simulink model "Main_simulation"  (R2021b)
settings: Solver=FixedStepAuto  StartTime=0.0  StopTime=Time  FixedStep=t_sample  RelTol=1e-13  AbsTol=1e-19
model workspace (MAT data in the model file):
  S_N = 0
values from neighbouring files (symbols this model uses):
  a = 8.6251e+06    (= 8625100)    [Main.m]    (also in main_code.m)
  A_BN_0 = [1/3, 2/3, 2/3;             2/3, 1/3, -2/3;            -2/3, 2/3,-1/3]    [Main.m]    (also in main_code.m = eye(3))
  A_rw = [1 0 0 1/sqrt(3);         0 1 0 1/sqrt(3) ... (first row only)    [Main.m]    (also in main_code.m)
  A_rw_star = [5/6 -1/6 -1/6;              -1/6  5/6 -1/6 ... (first row only)    [Main.m]    (also in main_code.m)
  acc_m = deg2rad(5)    [main_code.m]
  acc_S = deg2rad(0.25)    [main_code.m]
  c = 299792*10^3    (= 299792000)    [Main.m]    (also in main_code.m)
  control = 2    [main_code.m]
  e = 0.1195    [Main.m]    (also in main_code.m)
  G = 6.67259 * 1e-11    (= 6.67259e-11)    [Main.m]    (also in main_code.m = [gn, gm, gvali, gsvi])
  H = [hn, hm, hvali, hsvi]    [main_code.m]
  i = 0.3815    [Main.m]    (also in main_code.m)
  MB = [2000; 0.3; 1; 0.12].*1e-2    [Main.m]    (also in main_code.m = [1; 0.3; 0.3; 0.3])
  mr = 1.2*1e-4    (= 0.00012)    [Main.m]    (also in main_code.m)
  mu_P = G * Mt    (= 398527110340000)    [main_code.m]
  omega_0 = [om_x, om_y, om_z]    [Main.m]    (also in main_code.m = [w_0x; w_0y; w_0z])
  rho_d_MB = 0.1    [Main.m]    (also in main_code.m)
  rho_d_SP = 0.1    [main_code.m]
  rho_s_MB = 0.5    [Main.m]    (also in main_code.m)
  rho_s_SP = 0.1    [main_code.m]
  sig_b = sig_b^2    [Main.m]    (also in main_code.m)
  sig_n = 0.15*pi/180/3600/sqrt(t_sample)    [Main.m]    (also in main_code.m)
  SP = [2000; 0.3; 1; 0.12].*1e-2    [Main.m]    (also in main_code.m = [3; 0.3; 1; 0.1])
  t_sample = 1/5    (= 0.2)    [Main.m]    (also in main_code.m = 0.1)
  theta0 = 0    [Main.m]
  theta_0 = 0    [main_code.m]
libraries: matrix_library x16, vrlib x8, simulink x2, simulink_extras x1
(part 1 of 4)
settings Model: Creator=adity  LastModifiedBy=adity
settings SolverCC: ZeroCrossControl=DisableAll
settings DebuggingCC: AlgebraicLoopMsg=none

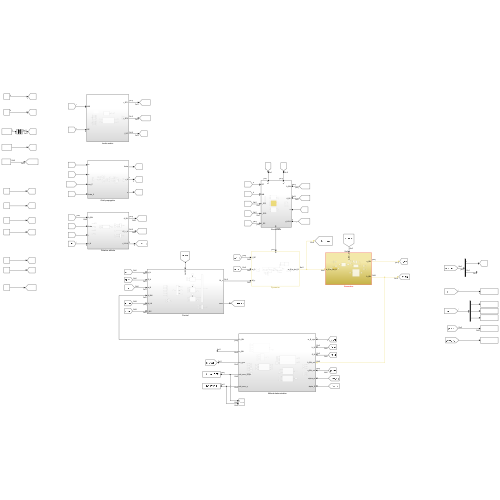
[thumbnail: Simulink's stored preview of the top-level diagram]
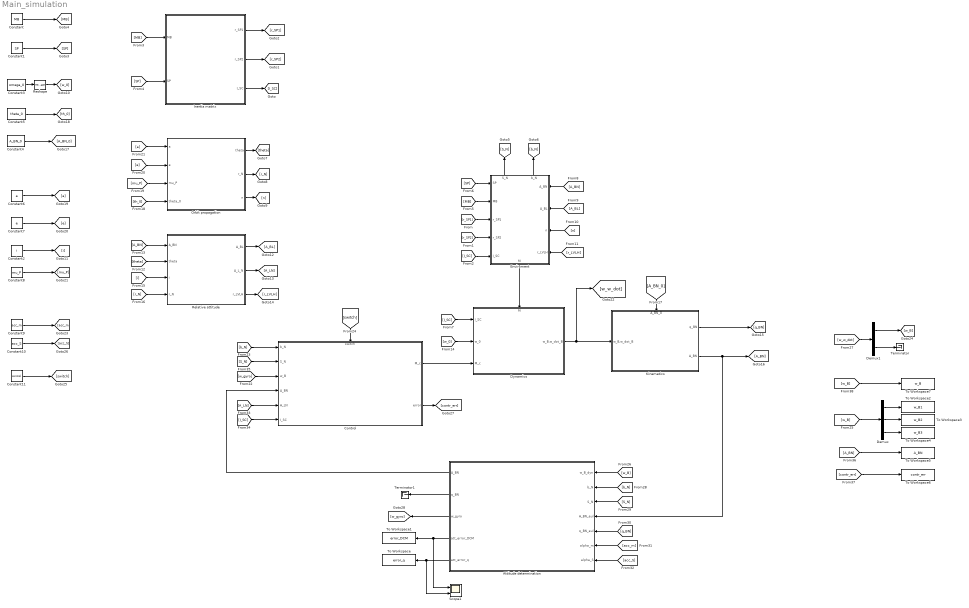
== system Main_simulation ==
  Attitude determination : Subsystem
  Constant : Constant  Value=MB
  Constant1 : Constant  Value=SP
  Constant10 : Constant  Value=acc_S
  Constant11 : Constant  Value=control
  Constant2 : Constant  Value=i
  Constant3 : Constant  Value=omega_0
  Constant4 : Constant  Value=A_BN_0
  Constant5 : Constant  Value=theta_0
  Constant6 : Constant  Value=a
  Constant7 : Constant  Value=e
  Constant8 : Constant  Value=mu_P
  Constant9 : Constant  Value=acc_m
  Control : Subsystem
      settings: PortSchema="{\"entries\":[{\"content\":{\"sides\":[{\"content\":{\"connectorIds\":[\"In1\",\"In2\",\"In3\",\"In4\",\"In5\",\"In6\"]},\"type\":\"ConnectorPlacement.EquallySpacedRectSide\",\"uuid\":\"def4633e-af2e-433f-a30d-e529dfff5b8a\"},{\"content\":{\"connectorIds\":[\"Out1\",\"Out2\"],\"side\":\"RIGHT\"},\"type\":\"ConnectorPlacement.EquallySpacedRectSide\",\"uuid\":\"7f0b35d9-01b3-48bb-a9b6-91939c0c12bf\"},{\"content\":{\"connectorIds\":[\"In7\"],\"side\":\"TOP\"},\"type\":\"ConnectorPlacement.EquallySpacedRectSide\",\"uuid\":\"2761e93e-9101-43c9-a9ad-74672a083719\"}]},\"type\":\"ConnectorPlacement.EquallySpacedConnector\",\"uuid\":\"8d28cc38-98df-4fe9-a975-1ea4168058d4\"}],\"packageUris\":[\"http://schema.mathworks.com/mf0/Connector/R2020b\"],\"version\":\"1.0\"}"
  Demux : Demux  Outputs=3
  Demux1 : Demux  Outputs=2
  Dynamics : Subsystem
      settings: PortSchema="{\"entries\":[{\"content\":{\"sides\":[{\"content\":{\"connectorIds\":[\"In1\",\"In2\",\"In3\"]},\"type\":\"ConnectorPlacement.EquallySpacedRectSide\",\"uuid\":\"0fb0fd28-732a-45b7-951f-4b0b2306202c\"},{\"content\":{\"connectorIds\":[\"Out1\"],\"side\":\"RIGHT\"},\"type\":\"ConnectorPlacement.EquallySpacedRectSide\",\"uuid\":\"160a6d95-5e8b-4088-9ac4-372e2ef53b1e\"},{\"content\":{\"connectorIds\":[\"In4\"],\"side\":\"TOP\"},\"type\":\"ConnectorPlacement.EquallySpacedRectSide\",\"uuid\":\"bc0d773d-9b3c-40c2-804a-fc9efd6e220c\"}]},\"type\":\"ConnectorPlacement.EquallySpacedConnector\",\"uuid\":\"1f85a25c-c8d4-4d9d-9994-483d99135538\"}],\"packageUris\":[\"http://schema.mathworks.com/mf0/Connector/R2020b\"],\"version\":\"1.0\"}"
  Enviroment : Subsystem
      settings: PortSchema="{\"entries\":[{\"content\":{\"sides\":[{\"content\":{\"connectorIds\":[\"Out2\",\"Out3\"]},\"type\":\"ConnectorPlacement.EquallySpacedRectSide\",\"uuid\":\"77a65197-c5ef-4c05-af97-bd670bb59a1b\"},{\"content\":{\"connectorIds\":[\"Out1\"],\"side\":\"RIGHT\"},\"type\":\"ConnectorPlacement.EquallySpacedRectSide\",\"uuid\":\"f4905732-994b-44e8-915f-1f1165b6d340\"},{\"content\":{\"connectorIds\":[\"In1\",\"In2\",\"In3\",\"In4\",\"In5\"],\"side\":\"TOP\"},\"type\":\"ConnectorPlacement.EquallySpacedRectSide\",\"uuid\":\"dbb628bc-072b-4daa-a580-a056bf799753\"},{\"content\":{\"connectorIds\":[\"In6\",\"In7\",\"In8\",\"In9\"],\"side\":\"BOTTOM\"},\"type\":\"ConnectorPlacement.EquallySpacedRectSide\",\"uuid\":\"e6af6235-b92e-4098-9bbc-91b77f168ead\"}]},\"type\":\"ConnectorPlacement.EquallySpacedConnector\",\"uuid\":\"a4645f0d-8f51-4ba7-9ec5-d423e83ccc17\"}],\"packageUris\":[\"http://schema.mathworks.com/mf0/Connector/R2020b\"],\"version\":\"1.0\"}"
  Inertia matrix : Subsystem
  Kinematics : Subsystem
      settings: PortSchema="{\"entries\":[{\"content\":{\"sides\":[{\"content\":{\"connectorIds\":[\"In1\"]},\"type\":\"ConnectorPlacement.EquallySpacedRectSide\",\"uuid\":\"b4580536-f47d-4a76-9d7a-ad9e45e6fd22\"},{\"content\":{\"connectorIds\":[\"Out1\",\"Out2\"],\"side\":\"RIGHT\"},\"type\":\"ConnectorPlacement.EquallySpacedRectSide\",\"uuid\":\"4273ed6e-d469-4a82-9e71-da4fb1c9f709\"},{\"content\":{\"connectorIds\":[\"In2\"],\"side\":\"TOP\"},\"type\":\"ConnectorPlacement.EquallySpacedRectSide\",\"uuid\":\"bac57a2b-a638-4d55-8f6f-550bb52319aa\"}]},\"type\":\"ConnectorPlacement.EquallySpacedConnector\",\"uuid\":\"29527554-7b77-4957-9d93-347c44cffae5\"}],\"packageUris\":[\"http://schema.mathworks.com/mf0/Connector/R2020b\"],\"version\":\"1.0\"}"
  Orbit propagation : Subsystem
  Relative attitude : Subsystem
  Reshape : Reshape  OutputDimensionality=Column vector (2-D)
  Scope1 : Scope  NumInputPorts=2
  Terminator : Terminator
  Terminator1 : Terminator
  To Workspace : ToWorkspace  VariableName=error_q  SaveFormat=Timeseries  SampleTime=-1
  To Workspace1 : ToWorkspace  VariableName=error_DCM  SaveFormat=Timeseries  SampleTime=-1
  To Workspace2 : ToWorkspace  VariableName=w_B1  SaveFormat=Timeseries  SampleTime=-1
  To Workspace3 : ToWorkspace  VariableName=w_B2  SaveFormat=Timeseries  SampleTime=-1
  To Workspace4 : ToWorkspace  VariableName=w_B3  SaveFormat=Timeseries  SampleTime=-1
  To Workspace5 : ToWorkspace  VariableName=A_BN  SaveFormat=Timeseries  SampleTime=-1
  To Workspace6 : ToWorkspace  VariableName=contr_err  SaveFormat=Timeseries  SampleTime=-1
  To Workspace7 : ToWorkspace  VariableName=w_B  SaveFormat=Timeseries  SampleTime=-1
  wires:
  Inertia matrix/3(I_SC) -> [I_SC]
  Inertia matrix/2(r_SP2) -> [r_SP2]
  Inertia matrix/1(r_SP1) -> [r_SP1]
  [r_SP1] -> Enviroment/3(r_SP1)
  [r_SP2] -> Enviroment/4(r_SP2)
  [I_SC] -> Enviroment/5(I_SC)
  Constant/1 -> [MB]
  Constant1/1 -> [SP]
  [MB] -> Inertia matrix/1(MB)
  [SP] -> Inertia matrix/2(SP)
  [MB] -> Enviroment/2(MB)
  [SP] -> Enviroment/1(SP)
  Enviroment/1(M) -> Dynamics/4(M)
  [I_SC] -> Dynamics/1(I_SC)
  Enviroment/2(S_N) -> [S_N]
  Enviroment/3(b_N) -> [b_N]
  [A_BN] -> Enviroment/6(A_BN)
  [A_BL] -> Enviroment/7(A_BL)
  [n] -> Enviroment/8(n)
  [r_LVLH] -> Enviroment/9(r_LVLH)
  Orbit propagation/1(theta) -> [theta]
  Orbit propagation/2(r_N) -> [r_N]
  Orbit propagation/3(n) -> [n]
  [theta] -> Relative attitude/2(theta)
  [A_BN] -> Relative attitude/1(A_BN)
  [w_0] -> Dynamics/2(w_0)
  Constant2/1 -> [i]
  [i] -> Relative attitude/3(i)
  Relative attitude/1(A_BL) -> [A_BL]
  Relative attitude/2(A_L_N) -> [A_LN]
  Dynamics/1(w_B,w_dot_B) -> Kinematics/1(w_B,w_dot_B), [w_w_dot]
  [r_N] -> Relative attitude/4(r_N)
  Relative attitude/3(r_LVLH) -> [r_LVLH]
  Kinematics/1(q_BN) -> [q_BN]
  Kinematics/2(A_BN) -> [A_BN], Attitude determination/4(A_BN_eul)
  [A_BN_0] -> Kinematics/2(A_BN_0)
  Constant4/1 -> [A_BN_0]
  Constant5/1 -> [th_0]
  [th_0] -> Orbit propagation/4(theta_0)
  Constant6/1 -> [a]
  Constant7/1 -> [e]
  Constant8/1 -> [mu_P]
  [mu_P] -> Orbit propagation/3(mu_P)
  [e] -> Orbit propagation/2(e)
  [a] -> Orbit propagation/1(a)
  [w_B] -> Demux/1
  Constant3/1 -> Reshape/1
  Reshape/1 -> [w_0]
  Demux1/1 -> [w_B]
  [w_w_dot] -> Demux1/1
  Demux1/2 -> Terminator/1
  [w_gyro] -> Control/3(w_B)
  [b_N] -> Control/1(b_N)
  [w_B] -> Attitude determination/1(w_B_dyn)
  [b_N] -> Attitude determination/2(b_N)
  [S_N] -> Attitude determination/3(S_N)
  [q_BN] -> Attitude determination/5(q_BN_eul)
  [acc_m] -> Attitude determination/6(alpha_m)
  Constant9/1 -> [acc_m]
  Constant10/1 -> [acc_S]
  [acc_S] -> Attitude determination/7(alpha_S)
  Attitude determination/5(att_error_q) -> Scope1/2, To Workspace/1
  Attitude determination/3(w_gyro) -> [w_gyro]
  [A_LN] -> Control/5(A_LN)
  [I_SC] -> Control/6(I_SC)
  Control/1(M_c) -> Dynamics/3(M_c)
  Demux/1 -> To Workspace2/1
  Demux/2 -> To Workspace3/1
  Demux/3 -> To Workspace4/1
  Constant11/1 -> [switch]
  [switch] -> Control/7(switch)
  Attitude determination/2(q_BN) -> Terminator1/1
  [S_N] -> Control/2(S_N)
  [A_BN] -> To Workspace5/1
  Control/2(error) -> [contr_err]
  [contr_err] -> To Workspace6/1
  [w_B] -> To Workspace7/1
  Attitude determination/1(A_BN) -> Control/4(A_BN)
  Attitude determination/4(att_error_DCM) -> Scope1/1, To Workspace1/1

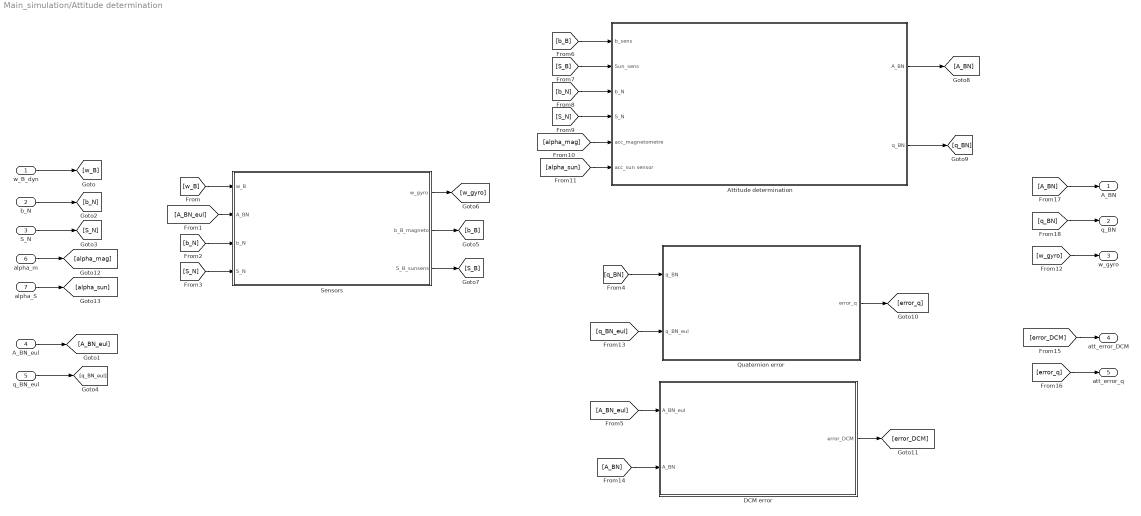
== system Main_simulation/Attitude determination ==
  w_B_dyn : Inport
  b_N : Inport  Port=2
  S_N : Inport  Port=3
  A_BN_eul : Inport  Port=4
  q_BN_eul : Inport  Port=5
  alpha_m : Inport  Port=6
  alpha_S : Inport  Port=7
  Attitude determination : Subsystem
  DCM error : Subsystem
  Quaternion error : Subsystem
  Sensors : Subsystem
  A_BN : Outport
  q_BN : Outport  Port=2
  w_gyro : Outport  Port=3
  att_error_DCM : Outport  Port=4
  att_error_q : Outport  Port=5
  wires:
  w_B_dyn/1 -> [w_B]
  A_BN_eul/1 -> [A_BN_eul]
  b_N/1 -> [b_N]
  S_N/1 -> [S_N]
  [w_B] -> Sensors/1(w_B)
  [A_BN_eul] -> Sensors/2(A_BN)
  [b_N] -> Sensors/3(b_N)
  [S_N] -> Sensors/4(S_N)
  q_BN_eul/1 -> [q_BN_eul]
  Sensors/2(b_B_magneto) -> [b_B]
  Sensors/1(w_gyro) -> [w_gyro]
  Sensors/3(S_B_sunsens) -> [S_B]
  [q_BN] -> Quaternion error/1(q_BN)
  [A_BN_eul] -> DCM error/1(A_BN_eul)
  [b_B] -> Attitude determination/1(b_sens)
  [S_B] -> Attitude determination/2(Sun_sens)
  [b_N] -> Attitude determination/3(b_N)
  [S_N] -> Attitude determination/4(S_N)
  [alpha_mag] -> Attitude determination/5(acc_magnetometre)
  [alpha_sun] -> Attitude determination/6(acc_sun sensor)
  [w_gyro] -> w_gyro/1
  [q_BN_eul] -> Quaternion error/2(q_BN_eul)
  [A_BN] -> DCM error/2(A_BN)
  Quaternion error/1(error_q) -> [error_q]
  DCM error/1(error_DCM) -> [error_DCM]
  [error_DCM] -> att_error_DCM/1
  [error_q] -> att_error_q/1
  [A_BN] -> A_BN/1
  [q_BN] -> q_BN/1
  alpha_m/1 -> [alpha_mag]
  alpha_S/1 -> [alpha_sun]
  Attitude determination/2(q_BN) -> [q_BN]
  Attitude determination/1(A_BN) -> [A_BN]

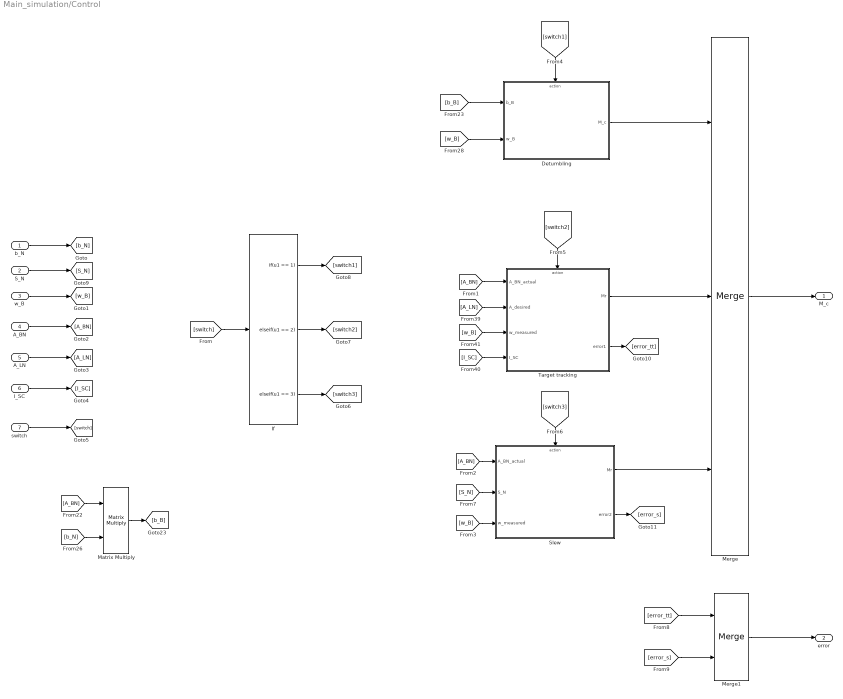
== system Main_simulation/Control ==
  b_N : Inport
  S_N : Inport  Port=2
  w_B : Inport  Port=3
  A_BN : Inport  Port=4
  A_LN : Inport  Port=5
  I_SC : Inport  Port=6
  switch : Inport  Port=7
  Detumbling : Subsystem  TreatAsAtomicUnit=on
  If : If  IfExpression=u1 == 1  ElseIfExpressions=u1 == 2, u1 == 3  ShowElse=off
  Matrix Multiply : Product  Multiplication=Matrix(*)
  Merge : Merge  Inputs=3
  Merge1 : Merge
  Slew : Subsystem  TreatAsAtomicUnit=on
  Target tracking : Subsystem  TreatAsAtomicUnit=on
  M_c : Outport
  error : Outport  Port=2
  wires:
  Matrix Multiply/1 -> [b_B]
  [b_N] -> Matrix Multiply/2
  [A_BN] -> Matrix Multiply/1
  [b_B] -> Detumbling/1(b_B)
  b_N/1 -> [b_N]
  w_B/1 -> [w_B]
  A_BN/1 -> [A_BN]
  Target tracking/1(Mr) -> Merge/2
  [A_LN] -> Target tracking/2(A_desired)
  [A_BN] -> Target tracking/1(A_BN_actual)
  [w_B] -> Target tracking/3(w_measured)
  A_LN/1 -> [A_LN]
  I_SC/1 -> [I_SC]
  [w_B] -> Detumbling/2(w_B)
  Merge/1 -> M_c/1
  Detumbling/1(M_c) -> Merge/1
  [I_SC] -> Target tracking/4(I_SC)
  [A_BN] -> Slew/1(A_BN_actual)
  [w_B] -> Slew/3(w_measured)
  switch/1 -> [switch]
  [switch] -> If/1
  If/3 -> [switch3]
  If/2 -> [switch2]
  If/1 -> [switch1]
  [switch1] -> Detumbling/Action
  [switch2] -> Target tracking/Action
  Slew/1(Mr) -> Merge/3
  S_N/1 -> [S_N]
  [S_N] -> Slew/2(S_N)
  [switch3] -> Slew/Action
  Target tracking/2(error1) -> [error_tt]
  Slew/2(error2) -> [error_s]
  [error_tt] -> Merge1/1
  [error_s] -> Merge1/2
  Merge1/1 -> error/1

== system Main_simulation/Dynamics ==
  I_SC : Inport
  w_0 : Inport  Port=2
  M_c : Inport  Port=3
  M : Inport  Port=4
  Add : Sum
  Cross Product : vrlib/Utilities/Cross Product
  Demux : Demux  Outputs=3
  Gain5 : Gain  Gain=-1
  Integrator4 : Integrator  InitialConditionSource=external  InitialCondition=omega_0
  Mux : Mux  Inputs=2
  Product6 : Product  Multiplication=Matrix(*)
  Product7 : Product  Multiplication=Matrix(*)
  Reciprocal : Product  Inputs=/  Multiplication=Matrix(*)
  Scope : Scope  NumInputPorts=3
  Scope1 : Scope
  Sum2 : Sum
  w_B,w_dot_B : Outport
  wires:
  Sum2/1 -> Product7/2
  Product6/1 -> Cross Product/2
  Product7/1 -> [w_dot_B], Integrator4/1
  Cross Product/1 -> Gain5/1
  Gain5/1 -> Sum2/1
  Integrator4/1 -> [w_B], Demux/1, Cross Product/1, Product6/2
  I_SC/1 -> [I_SC]
  [I_SC] -> Product6/1
  [I_SC] -> Reciprocal/1
  Reciprocal/1 -> Product7/1
  w_0/1 -> [w_0]
  [w_0] -> Integrator4/2
  Demux/2 -> Scope/2  "om_y"
  Demux/1 -> Scope/1  "om_x"
  Demux/3 -> Scope/3  "om_z"
  Add/1 -> Sum2/2
  Mux/1 -> w_B,w_dot_B/1
  [w_B] -> Mux/1
  [w_dot_B] -> Mux/2
  M/1 -> Add/1, Scope1/1
  M_c/1 -> Add/2

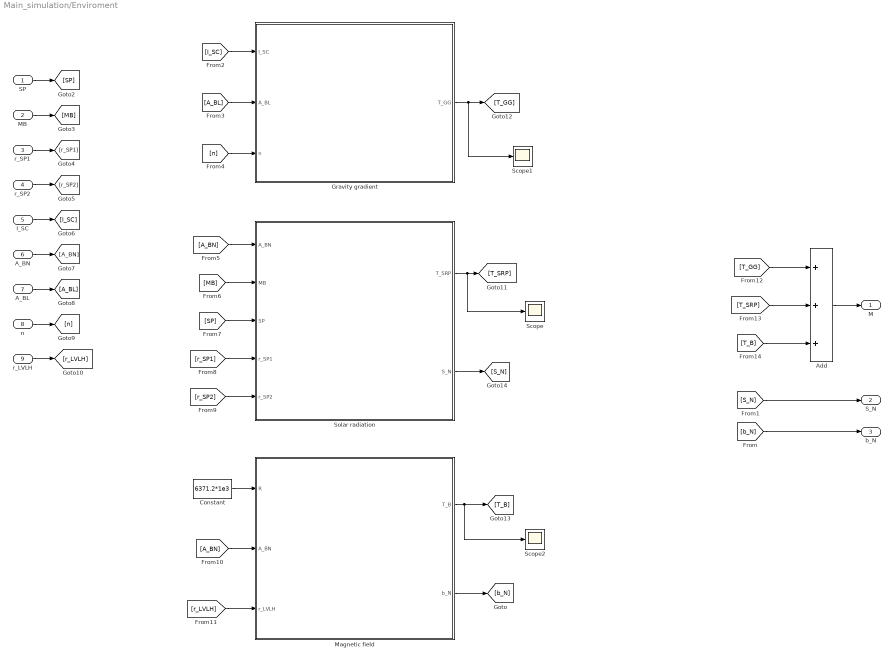
== system Main_simulation/Enviroment ==
  SP : Inport
  MB : Inport  Port=2
  r_SP1 : Inport  Port=3
  r_SP2 : Inport  Port=4
  I_SC : Inport  Port=5
  A_BN : Inport  Port=6
  A_BL : Inport  Port=7
  n : Inport  Port=8
  r_LVLH : Inport  Port=9
  Add : Sum  Inputs=+++
  Constant : Constant  Value=6371.2*1e3
  Gravity gradient : Subsystem
  Magnetic field : Subsystem
  Scope : Scope
  Scope1 : Scope
  Scope2 : Scope
  Solar radiation : Subsystem
  M : Outport
  S_N : Outport  Port=2
  b_N : Outport  Port=3
  wires:
  Add/1 -> M/1
  Constant/1 -> Magnetic field/1(R)
  [b_N] -> b_N/1
  [S_N] -> S_N/1
  SP/1 -> [SP]
  MB/1 -> [MB]
  r_SP1/1 -> [r_SP1]
  r_SP2/1 -> [r_SP2]
  I_SC/1 -> [I_SC]
  A_BN/1 -> [A_BN]
  A_BL/1 -> [A_BL]
  n/1 -> [n]
  r_LVLH/1 -> [r_LVLH]
  Magnetic field/2(b_N) -> [b_N]
  Solar radiation/1(T_SRP) -> Scope/1, [T_SRP]
  Gravity gradient/1(T_GG) -> Scope1/1, [T_GG]
  Magnetic field/1(T_B) -> Scope2/1, [T_B]
  [I_SC] -> Gravity gradient/1(I_SC)
  [A_BL] -> Gravity gradient/2(A_BL)
  [n] -> Gravity gradient/3(n)
  [A_BN] -> Solar radiation/1(A_BN)
  [MB] -> Solar radiation/2(MB)
  [SP] -> Solar radiation/3(SP)
  [r_SP1] -> Solar radiation/4(r_SP1)
  [r_SP2] -> Solar radiation/5(r_SP2)
  [A_BN] -> Magnetic field/2(A_BN)
  [r_LVLH] -> Magnetic field/3(r_LVLH)
  Solar radiation/2(S_N) -> [S_N]
  [T_GG] -> Add/1
  [T_SRP] -> Add/2
  [T_B] -> Add/3

== system Main_simulation/Inertia matrix ==
  note: a long side, b middle side h short side
      | long side on x axis solar panel
      | middle side z axis solar panel
      | long side y axis main body
      | middle side x axis main body
      | short side z axis main body
  MB : Inport
  SP : Inport  Port=2
  Constant : Constant  Value=[19.5 0 0; 0 19 0; 0 0 12.6]  VectorParams1D=off
  Demux : Demux
  Demux1 : Demux
  Reshape : Reshape  OutputDimensionality=Customize  OutputDimensions=[3,3]
  Terminator{,1..5} (6 alike) : Terminator
  r_SP : Subsystem
  r_SP1 : Outport
  r_SP2 : Outport  Port=2
  I_SC : Outport  Port=3
  wires:
  MB/1 -> Demux1/1
  Demux/1 -> Terminator5/1
  r_SP/1(r_SP1) -> [r_SP1]
  [r_SP1] -> r_SP1/1
  [r_SP2] -> r_SP2/1
  r_SP/2(r_SP2) -> [r_SP2]
  Demux/2 -> Terminator4/1
  Demux/3 -> [b_SP]
  Demux/4 -> Terminator3/1
  [b_SP] -> r_SP/1(b_SP)
  Demux1/4 -> Terminator1/1
  Demux1/3 -> Terminator/1
  Demux1/2 -> [a_MB]
  Demux1/1 -> Terminator2/1
  [a_MB] -> r_SP/2(a_MB)
  SP/1 -> Demux/1
  [I_SC] -> I_SC/1
  Constant/1 -> Reshape/1
  Reshape/1 -> [I_SC]

== system Main_simulation/Kinematics ==
  w_B,w_dot_B : Inport
  A_BN_0 : Inport  Port=2
  DCM to quaternion : Subsystem
  Demux : Demux  Outputs=2
  Gain : Gain  Gain=1/2
  Integrator : Integrator  InitialConditionSource=external  InitialCondition=[0; 0; 0; 1]
  Matrix Multiply : Product  Multiplication=Matrix(*)
  Normalisation : Subsystem
  Reshape : Reshape  OutputDimensionality=Column vector (2-D)
  Subsystem : Subsystem
  Terminator : Terminator
  q to DCM : Subsystem
  q_BN : Outport
  A_BN : Outport  Port=2
  wires:
  w_B,w_dot_B/1 -> Demux/1
  Demux/1 -> [w_B]
  Demux/2 -> Terminator/1
  A_BN_0/1 -> [A_BN_0]
  [q_0] -> Integrator/2
  [w_B] -> Subsystem/1(w_B)
  DCM to quaternion/1(q) -> [q_0]
  Subsystem/1(OMEGA) -> [OMEGA]
  Reshape/1 -> Normalisation/1(In1)
  Integrator/1 -> Reshape/1  "q(t)"
  [OMEGA] -> Gain/1
  Gain/1 -> Matrix Multiply/1
  Normalisation/1(Out1) -> Matrix Multiply/2, [q_BN]  "q(t)"
  Matrix Multiply/1 -> Integrator/1  "dq/dt"
  [A_BN_0] -> DCM to quaternion/1(DCM)
  [q_BN] -> q_BN/1
  [A_BN] -> A_BN/1
  q to DCM/1(A_BN) -> [A_BN]
  [q_BN] -> q to DCM/1(q_BN)

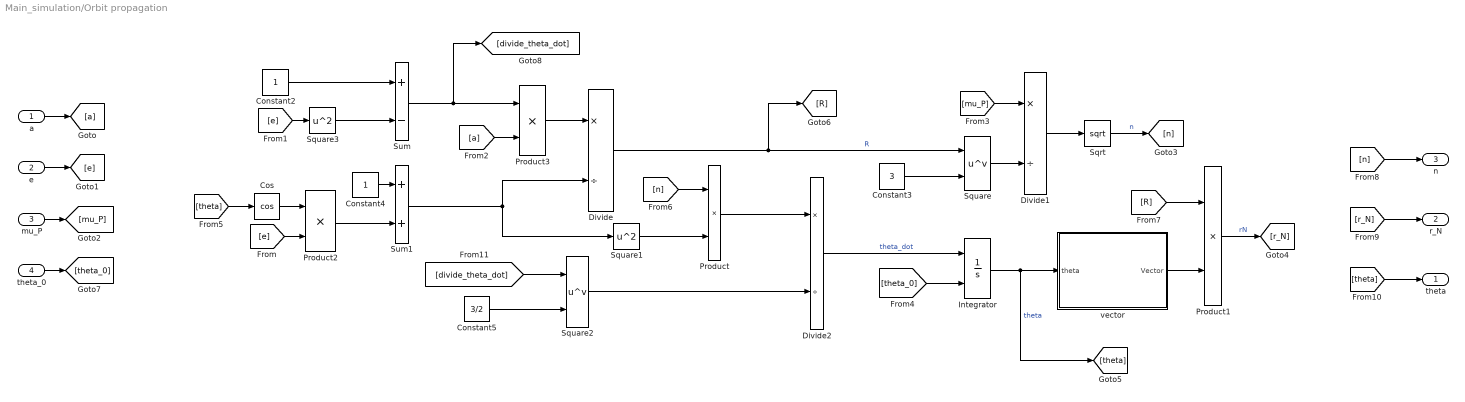
== system Main_simulation/Orbit propagation ==
  a : Inport
  e : Inport  Port=2
  mu_P : Inport  Port=3
  theta_0 : Inport  Port=4
  Constant2 : Constant
  Constant3 : Constant  Value=3
  Constant4 : Constant
  Constant5 : Constant  Value=3/2
  Cos : Trigonometry  Operator=cos
  Divide : Product  Inputs=*/
  Divide1 : Product  Inputs=*/
  Divide2 : Product  Inputs=*/
  Integrator : Integrator  InitialConditionSource=external  InitialCondition=theta0
  Product{,1..3} (4 alike) : Product
  Sqrt : Sqrt  SaturateOnIntegerOverflow=on
  Square : Math  Operator=pow  SaturateOnIntegerOverflow=on
  Square1 : Math  Operator=square  SaturateOnIntegerOverflow=on
  Square2 : Math  Operator=pow  SaturateOnIntegerOverflow=on
  Square3 : Math  Operator=square  SaturateOnIntegerOverflow=on
  Sum : Sum  Inputs=+-
  Sum1 : Sum
  vector : Subsystem
  theta : Outport
  r_N : Outport  Port=2
  n : Outport  Port=3
  wires:
  Constant2/1 -> Sum/1
  Square3/1 -> Sum/2
  Sum/1 -> [divide_theta_dot], Product3/1
  Product3/1 -> Divide/1
  Constant4/1 -> Sum1/1
  Sum1/1 -> Square1/1, Divide/2
  Product2/1 -> Sum1/2
  Cos/1 -> Product2/1
  Integrator/1 -> [theta], vector/1(theta)  "theta"
  Divide1/1 -> Sqrt/1
  [mu_P] -> Divide1/1
  Square/1 -> Divide1/2
  Divide/1 -> [R], Square/1  "R"
  Constant3/1 -> Square/2
  Sqrt/1 -> [n]  "n"
  Square1/1 -> Product/2
  Constant5/1 -> Square2/2
  Product/1 -> Divide2/1
  Divide2/1 -> Integrator/1  "theta_dot"
  vector/1(Vector) -> Product1/2
  Square2/1 -> Divide2/2
  a/1 -> [a]
  e/1 -> [e]
  mu_P/1 -> [mu_P]
  [e] -> Product2/2
  [e] -> Square3/1
  [a] -> Product3/2
  [theta_0] -> Integrator/2
  Product1/1 -> [r_N]  "rN"
  [theta] -> Cos/1
  [n] -> Product/1
  [R] -> Product1/1
  [n] -> n/1
  [r_N] -> r_N/1
  [theta] -> theta/1
  theta_0/1 -> [theta_0]
  [divide_theta_dot] -> Square2/1

== system Main_simulation/Relative attitude ==
  A_BN : Inport
  theta : Inport  Port=2
  i : Inport  Port=3
  r_N : Inport  Port=4
  A_LN : Subsystem
  MatrixMultiply : Product  Multiplication=Matrix(*)
  MatrixMultiply1 : Product  Multiplication=Matrix(*)
  Transpose : Math  Operator=transpose  SaturateOnIntegerOverflow=on
  A_BL : Outport
  A_L_N : Outport  Port=2
  r_LVLH : Outport  Port=3
  wires:
  Transpose/1 -> MatrixMultiply/2
  MatrixMultiply/1 -> A_BL/1  "A_BL"
  theta/1 -> [theta]
  A_BN/1 -> [A_BN]
  [theta] -> A_LN/1(theta)
  A_LN/1(A_L_N) -> [A_LN]
  [i] -> A_LN/2(i)
  i/1 -> [i]
  [A_BN] -> MatrixMultiply/1
  [A_LN] -> Transpose/1
  [A_LN] -> A_L_N/1
  MatrixMultiply1/1 -> r_LVLH/1  "A_BL"
  [A_LN] -> MatrixMultiply1/1
  r_N/1 -> [r_N]
  [r_N] -> MatrixMultiply1/2

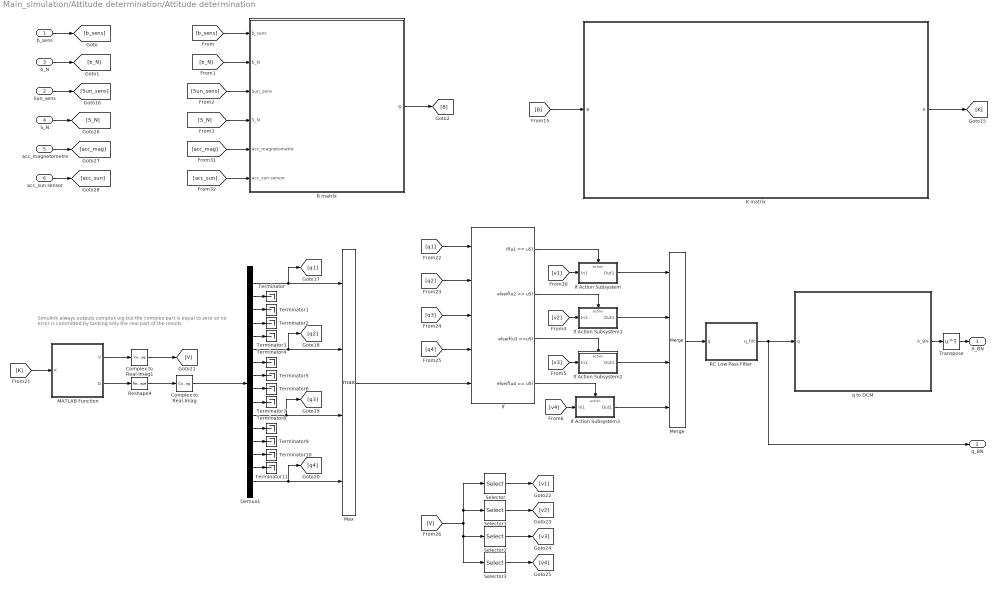
== system Main_simulation/Attitude determination/Attitude determination ==
  note: Simulink always outputs complex eig but the complex part is equal to zero so
      | no error is committed by tanking only the real part of the results
  b_sens : Inport
  Sun_sens : Inport  Port=2
  b_N : Inport  Port=3
  S_N : Inport  Port=4
  acc_magnetometre : Inport  Port=5
  acc_sun sensor : Inport  Port=6
  B matrix : Subsystem
  Complex to Real-Imag : ComplexToRealImag  Output=Real
  Complex to Real-Imag1 : ComplexToRealImag  Output=Real
  Demux1 : Demux  Outputs=16
  If : If  NumInputs=5  IfExpression=u1 == u5  ElseIfExpressions=u2 == u5, u3 ==u5, u4 == u5  ShowElse=off
  If Action Subsystem : Subsystem  TreatAsAtomicUnit=on
  If Action Subsystem1 : Subsystem  TreatAsAtomicUnit=on
  If Action Subsystem2 : Subsystem  TreatAsAtomicUnit=on
  If Action Subsystem3 : Subsystem  TreatAsAtomicUnit=on
  K matrix : Subsystem
  MATLAB Function : MATLAB Function  TreatAsAtomicUnit=on
  Max : MinMax  Function=max  Inputs=4
  Merge : Merge  Inputs=4
  RC Low Pass FIlter : Subsystem
  Reshape4 : Reshape  OutputDimensionality=Column vector (2-D)
  Selector : Selector  NumberOfDimensions=2  InputPortWidth=3  IndexOptions=Index vector (dialog),Index vector (dialog)  Indices=[1 2 3 4],1  OutputSizes=1,1
  Selector1 : Selector  NumberOfDimensions=2  InputPortWidth=3  IndexOptions=Index vector (dialog),Index vector (dialog)  Indices=[1 2 3 4],2  OutputSizes=1,1
  Selector2 : Selector  NumberOfDimensions=2  InputPortWidth=3  IndexOptions=Index vector (dialog),Index vector (dialog)  Indices=[1 2 3 4],3  OutputSizes=1,1
  Selector3 : Selector  NumberOfDimensions=2  InputPortWidth=3  IndexOptions=Index vector (dialog),Index vector (dialog)  Indices=[1 2 3 4],4  OutputSizes=1,1
  Terminator{,1..11} (12 alike) : Terminator
  Transpose : Math  Operator=transpose  SaturateOnIntegerOverflow=on
  q to DCM : Subsystem
  A_BN : Outport
  q_BN : Outport  Port=2
  wires:
  MATLAB Function/2(D) -> Reshape4/1
  Demux1/2 -> Terminator/1
  Demux1/3 -> Terminator1/1
  Demux1/4 -> Terminator2/1
  Demux1/5 -> Terminator3/1
  Demux1/6 -> [q2], Max/2
  Demux1/7 -> Terminator4/1
  Demux1/8 -> Terminator5/1
  Demux1/9 -> Terminator6/1
  Demux1/10 -> Terminator7/1
  Demux1/11 -> [q3], Max/3
  Demux1/16 -> [q4], Max/4
  Demux1/12 -> Terminator8/1
  Demux1/13 -> Terminator9/1
  Demux1/14 -> Terminator10/1
  Demux1/15 -> Terminator11/1
  Reshape4/1 -> Complex to Real-Imag/1
  Max/1 -> If/5
  Demux1/1 -> [q1], Max/1
  [q1] -> If/1
  [q2] -> If/2
  [q4] -> If/4
  [q3] -> If/3
  MATLAB Function/1(V) -> Complex to Real-Imag1/1
  Selector1/1 -> [v2]
  Selector3/1 -> [v4]
  Selector2/1 -> [v3]
  Selector/1 -> [v1]
  [V] -> Selector/1, Selector1/1, Selector3/1, Selector2/1
  If/1 -> If Action Subsystem/Action
  If Action Subsystem/1(Out1) -> Merge/1
  If Action Subsystem3/1(Out1) -> Merge/4
  If Action Subsystem2/1(Out1) -> Merge/3
  If Action Subsystem1/1(Out1) -> Merge/2
  [v1] -> If Action Subsystem/1(In1)
  Complex to Real-Imag/1 -> Demux1/1
  Complex to Real-Imag1/1 -> [V]
  [K] -> MATLAB Function/1(K)
  B matrix/1(B) -> [B]
  b_N/1 -> [b_N]
  S_N/1 -> [S_N]
  acc_magnetometre/1 -> [acc_mag]
  acc_sun sensor/1 -> [acc_sun]
  [b_sens] -> B matrix/1(b_sens)
  [b_N] -> B matrix/2(b_N)
  [Sun_sens] -> B matrix/3(Sun_sens)
  [S_N] -> B matrix/4(S_N)
  [acc_mag] -> B matrix/5(acc_magnetometre)
  [acc_sun] -> B matrix/6(acc_sun sensor)
  [B] -> K matrix/1(B)
  K matrix/1(K) -> [K]
  Sun_sens/1 -> [Sun_sens]
  b_sens/1 -> [b_sens]
  q to DCM/1(A_BN) -> Transpose/1
  Merge/1 -> RC Low Pass FIlter/1(q)
  [v2] -> If Action Subsystem1/1(In1)
  If/2 -> If Action Subsystem1/Action
  If/3 -> If Action Subsystem2/Action
  [v3] -> If Action Subsystem2/1(In1)
  [v4] -> If Action Subsystem3/1(In1)
  If/4 -> If Action Subsystem3/Action
  RC Low Pass FIlter/1(q_filt) -> q_BN/1, q to DCM/1(q)
  Transpose/1 -> A_BN/1

== system Main_simulation/Attitude determination/DCM error ==
  A_BN_eul : Inport
  A_BN : Inport  Port=2
  Add : Sum  Inputs=+-
  Constant : Constant  Value=[1 0 0; 0 1 0; 0 0 1]
  Matrix Multiply : Product  Multiplication=Matrix(*)
  Reshape : Reshape  OutputDimensionality=Customize  OutputDimensions=[3,3]
  Transpose : Math  Operator=transpose  SaturateOnIntegerOverflow=on
  error_DCM : Outport
  wires:
  A_BN_eul/1 -> Transpose/1
  Transpose/1 -> Matrix Multiply/2
  A_BN/1 -> Matrix Multiply/1
  Add/1 -> error_DCM/1
  Matrix Multiply/1 -> Add/1
  Constant/1 -> Reshape/1
  Reshape/1 -> Add/2

== system Main_simulation/Attitude determination/Quaternion error ==
  q_BN : Inport
  q_BN_eul : Inport  Port=2
  Matrix Multiply : Product  Multiplication=Matrix(*)
  Q matrix : Subsystem
  q_vect : Selector  InputPortWidth=4  IndexOptions=Index vector (dialog)  Indices=[1 2 3]  OutputSizes=1
  error_q : Outport
  wires:
  q_BN/1 -> [q_att]
  q_BN_eul/1 -> [q_eul]
  [q_eul] -> Q matrix/1(q_eul)
  [q_att] -> Matrix Multiply/2
  Q matrix/1(Q_eul) -> Matrix Multiply/1
  Matrix Multiply/1 -> q_vect/1
  q_vect/1 -> error_q/1

== system Main_simulation/Attitude determination/Sensors ==
  w_B : Inport
  A_BN : Inport  Port=2
  b_N : Inport  Port=3
  S_N : Inport  Port=4
  Gyroscopes : Subsystem
  Magnetometer : Subsystem
  Sun sensor : Subsystem
  Zero-Order Hold{,1..3} (4 alike) : ZeroOrderHold  SampleTime=t_sample
  w_gyro : Outport
  b_B_magneto : Outport  Port=2
  S_B_sunsens : Outport  Port=3
  wires:
  [w_B] -> Gyroscopes/1(omega)
  [A_BN] -> Magnetometer/1(A_BN)
  [A_BN] -> Sun sensor/2(A_BN)
  Gyroscopes/1(w_gyro) -> [w_gyro]
  Magnetometer/1(b_B) -> [b_B]
  Sun sensor/1(S_B) -> [S_B]
  [w_gyro] -> w_gyro/1
  [b_B] -> b_B_magneto/1
  [S_B] -> S_B_sunsens/1
  w_B/1 -> Zero-Order Hold/1
  A_BN/1 -> Zero-Order Hold1/1
  b_N/1 -> Zero-Order Hold2/1
  S_N/1 -> Zero-Order Hold3/1
  [S_N] -> Sun sensor/1(S_N)
  [b_N] -> Magnetometer/2(b_N)
  Zero-Order Hold/1 -> [w_B]
  Zero-Order Hold1/1 -> [A_BN]
  Zero-Order Hold2/1 -> [b_N]
  Zero-Order Hold3/1 -> [S_N]

== system Main_simulation/Control/Detumbling ==
  b_B : Inport
  w_B : Inport  Port=2
  Action Port : ActionPort  ActionPortLabel=if(u1 == 1)
  Cross Product : matrix_library/Cross Product
      settings: SourceProductBaseCode=SL
  Cross Product1 : matrix_library/Cross Product
      settings: SourceProductBaseCode=SL
  Divide : Product  Inputs=/*
  Dot Product : DotProduct  InputSameDT=on  OutDataTypeStr=Inherit: Inherit via internal rule
  Gain : Gain  Gain=-1
  Product : Product
  k : Constant  Value=3.5e-2
  M_c : Outport
  wires:
  [b_B] -> Dot Product/2, Dot Product/1
  Product/1 -> Cross Product1/1
  Gain/1 -> Product/2
  Dot Product/1 -> Divide/1
  Divide/1 -> Product/1
  [b_B] -> Cross Product1/2
  b_B/1 -> [b_B]
  Cross Product/1 -> Divide/2
  [b_B] -> Cross Product/1
  w_B/1 -> [w_B]
  k/1 -> Gain/1
  Cross Product1/1 -> M_c/1
  [w_B] -> Cross Product/2

== system Main_simulation/Control/Slew ==
  A_BN_actual : Inport
  S_N : Inport  Port=2
  w_measured : Inport  Port=3
  Action Port : ActionPort  ActionPortLabel=elseif( u1 == 3)
  Demux : Demux  Outputs=3
  Desired attitude : Subsystem
  Gain : Gain  Gain=-1
  Gain1 : Gain  Gain=-1
  Matrix Multiply : Product  Multiplication=Matrix(*)
  Mux : Mux  Inputs=3
  Product : Product
  Product1 : Product
  Reaction wheel : Subsystem
  Reshape : Reshape  OutputDimensionality=Customize  OutputDimensions=[3,1]
  Reshape1 : Reshape  OutputDimensionality=Column vector (2-D)
  Reshape2 : Reshape  OutputDimensionality=Column vector (2-D)
  Scope{,1..3} (4 alike) : Scope
  Selector : Selector  NumberOfDimensions=2  InputPortWidth=3  IndexOptions=Index vector (dialog),Index vector (dialog)  Indices=2,1  OutputSizes=1,1
  Selector1 : Selector  NumberOfDimensions=2  InputPortWidth=3  IndexOptions=Index vector (dialog),Index vector (dialog)  Indices=3,1  OutputSizes=1,1
  Selector2 : Selector  NumberOfDimensions=2  InputPortWidth=3  IndexOptions=Index vector (dialog),Index vector (dialog)  Indices=3,2  OutputSizes=1,1
  Sum : Sum  Inputs=|+|-|
  Sum1 : Sum  Inputs=|+|+|
  Terminator : Terminator
  Terminator1 : Terminator
  Transpose : Math  Operator=transpose  SaturateOnIntegerOverflow=on
  Transpose1 : Math  Operator=transpose  SaturateOnIntegerOverflow=on
  k1 : Constant  Value=9.99e-2
  k2 : Constant  Value=1.25e-3
  Mr : Outport
  error2 : Outport  Port=2
  wires:
  Product/1 -> Reshape1/1
  Transpose1/1 -> Sum/1
  Selector1/1 -> Mux/2
  Reshape2/1 -> Sum1/1
  Sum/1 -> Selector1/1, Selector/1, Selector2/1
  Demux/3 -> Terminator1/1
  Selector2/1 -> Mux/3
  Matrix Multiply/1 -> Transpose1/1, Sum/2
  k2/1 -> Gain/1
  Reshape1/1 -> Sum1/2
  Mux/1 -> Reshape/1, Demux/1, Scope/1
  Sum1/1 -> Reaction wheel/1(Mc), Scope2/1
  k1/1 -> Gain1/1
  Product1/1 -> Reshape2/1
  Transpose/1 -> Matrix Multiply/2
  Gain1/1 -> Product/2
  Selector/1 -> Mux/1
  Demux/1 -> error2/1
  Reshape/1 -> Product1/1
  Demux/2 -> Terminator/1
  Gain/1 -> Product1/2
  Reaction wheel/1(Mr) -> Mr/1
  [w_B] -> Reaction wheel/2(w)
  A_BN_actual/1 -> [A_BN]
  [A_BN] -> Matrix Multiply/1
  [A_BN] -> Scope1/1
  Desired attitude/1(Desired A_BN) -> Transpose/1
  S_N/1 -> [S_N]
  w_measured/1 -> [w_B]
  [w_B] -> Scope3/1
  [w_B] -> Product/1
  [S_N] -> Desired attitude/1(S_N)

== system Main_simulation/Control/Target tracking ==
  A_BN_actual : Inport
  A_desired : Inport  Port=2
  w_measured : Inport  Port=3
  I_SC : Inport  Port=4
  Action Port : ActionPort  ActionPortLabel=elseif(u1 == 2)
  Cross Product : matrix_library/Cross Product
      settings: SourceProductBaseCode=SL
  Demux : Demux  Outputs=3
  Gain : Gain  Gain=-1
  Gain1 : Gain  Gain=-1
  Matrix Multiply : Product  Multiplication=Matrix(*)
  Matrix Multiply1 : Product  Multiplication=Matrix(*)
  Mux : Mux  Inputs=3
  Product : Product
  Product1 : Product
  Reaction wheel : Subsystem
  Reshape : Reshape  OutputDimensionality=Customize  OutputDimensions=[3,1]
  Reshape1 : Reshape  OutputDimensionality=Column vector (2-D)
  Reshape2 : Reshape  OutputDimensionality=Column vector (2-D)
  Scope : Scope
  Scope1 : Scope
  Scope4 : Scope
  Selector : Selector  NumberOfDimensions=2  InputPortWidth=3  IndexOptions=Index vector (dialog),Index vector (dialog)  Indices=2,1  OutputSizes=1,1
  Selector1 : Selector  NumberOfDimensions=2  InputPortWidth=3  IndexOptions=Index vector (dialog),Index vector (dialog)  Indices=3,1  OutputSizes=1,1
  Selector2 : Selector  NumberOfDimensions=2  InputPortWidth=3  IndexOptions=Index vector (dialog),Index vector (dialog)  Indices=3,2  OutputSizes=1,1
  Sum : Sum  Inputs=|+|-|
  Sum1 : Sum  Inputs=|+|+|+|
  Terminator : Terminator
  Terminator1 : Terminator
  Transpose : Math  Operator=transpose  SaturateOnIntegerOverflow=on
  Transpose1 : Math  Operator=transpose  SaturateOnIntegerOverflow=on
  k1 : Constant  Value=9.99e-2
  k2 : Constant  Value=1.5e-3
  Mr : Outport
  error1 : Outport  Port=2
  wires:
  Demux/1 -> error1/1
  Mux/1 -> Scope/1, Demux/1, Reshape/1
  A_BN_actual/1 -> Scope1/1, Matrix Multiply/1
  w_measured/1 -> [w_B]
  I_SC/1 -> [I_mat]
  Demux/3 -> Terminator1/1
  Matrix Multiply1/1 -> Cross Product/2
  Product/1 -> Reshape1/1
  Cross Product/1 -> Sum1/3
  k2/1 -> Gain/1
  k1/1 -> Gain1/1
  Matrix Multiply/1 -> Sum/2, Transpose1/1
  [I_mat] -> Matrix Multiply1/1
  Gain/1 -> Product1/2
  Reshape1/1 -> Sum1/2
  Transpose/1 -> Matrix Multiply/2
  Reshape/1 -> Product1/1
  Selector1/1 -> Mux/2
  Selector2/1 -> Mux/3
  Reshape2/1 -> Sum1/1
  Demux/2 -> Terminator/1
  A_desired/1 -> Scope4/1, Transpose/1
  Sum/1 -> Selector2/1, Selector/1, Selector1/1
  Transpose1/1 -> Sum/1
  Selector/1 -> Mux/1
  Gain1/1 -> Product/2
  Product1/1 -> Reshape2/1
  [w_B] -> Reaction wheel/2(w)
  Sum1/1 -> Reaction wheel/1(Mc)
  Reaction wheel/1(Mr) -> Mr/1
  [w_B] -> Product/1
  [w_B] -> Matrix Multiply1/2
  [w_B] -> Cross Product/1

== system Main_simulation/Enviroment/Gravity gradient ==
  I_SC : Inport
  A_BL : Inport  Port=2
  n : Inport  Port=3
  Constant : Constant  Value=3
  Constant1 : Constant  Value=[1 0 0]
  Demux : Demux  Outputs=9
  Demux1 : Demux  Outputs=3
  Matrix Multiply : Product  Multiplication=Matrix(*)
  Mux : Mux  Inputs=3
  Product{,1..9} (10 alike) : Product
  Reshape : Reshape  OutputDimensionality=Column vector (2-D)
  Reshape1 : Reshape  OutputDimensionality=Column vector (2-D)
  Reshape2 : Reshape  OutputDimensionality=Column vector (2-D)
  Scope : Scope  NumInputPorts=3
  Square : Math  Operator=square  SaturateOnIntegerOverflow=on
  Sum : Sum  Inputs=+-
  Sum1 : Sum  Inputs=+-
  Sum2 : Sum  Inputs=+-
  Terminator{,1..5} (6 alike) : Terminator
  T_GG : Outport
  wires:
  Demux/4 -> Terminator2/1
  Demux1/1 -> Product5/2, Product7/2
  Demux/2 -> Terminator/1
  Product6/1 -> Product9/1
  Sum/1 -> Product1/1
  Product1/1 -> Product6/1
  Demux/7 -> Terminator4/1
  Demux1/3 -> Product6/2, Product8/2
  Demux/1 -> Sum1/1
  Product5/1 -> Product8/1
  Demux/3 -> Terminator1/1
  I_SC/1 -> Reshape1/1
  Matrix Multiply/1 -> Demux1/1
  Demux/9 -> Sum2/2, Sum1/2, Sum/1
  Constant1/1 -> Reshape/1
  Sum1/1 -> Product2/1
  Sum2/1 -> Product3/1
  Product7/1 -> Scope/3, Mux/3
  Mux/1 -> Reshape2/1
  Demux/5 -> Sum/2, Sum2/1
  Demux/8 -> Terminator5/1
  A_BL/1 -> Matrix Multiply/1
  Product4/1 -> Product7/1
  Product8/1 -> Scope/2, Mux/2
  Demux/6 -> Terminator3/1
  Demux1/2 -> Product4/2, Product9/2
  Product2/1 -> Product5/1
  Product9/1 -> Scope/1, Mux/1
  Product3/1 -> Product4/1
  Reshape/1 -> Matrix Multiply/2
  Reshape1/1 -> Demux/1
  Reshape2/1 -> T_GG/1
  Square/1 -> Product/1
  Product/1 -> Product2/2, Product1/2, Product3/2
  Constant/1 -> Product/2
  n/1 -> Square/1

== system Main_simulation/Enviroment/Magnetic field ==
  R : Inport
  A_BN : Inport  Port=2
  r_LVLH : Inport  Port=3
  Cross Product : matrix_library/Cross Product
      settings: SourceProductBaseCode=SL
  b_B : Subsystem
  parasitic torque : Subsystem
  T_B : Outport
  b_N : Outport  Port=2
  wires:
  parasitic torque/1(m_par) -> [m_par]
  b_B/1(b_B) -> [b_B]
  b_B/2(b_N) -> [b_N]
  [m_par] -> Cross Product/1
  [b_B] -> Cross Product/2
  [b_N] -> b_N/1
  A_BN/1 -> [A_BN]
  R/1 -> [R]
  r_LVLH/1 -> [r_LVLH]
  [A_BN] -> b_B/1(A_BN)
  [R] -> b_B/2(R)
  [r_LVLH] -> b_B/3(r_LVLH)
  Cross Product/1 -> T_B/1

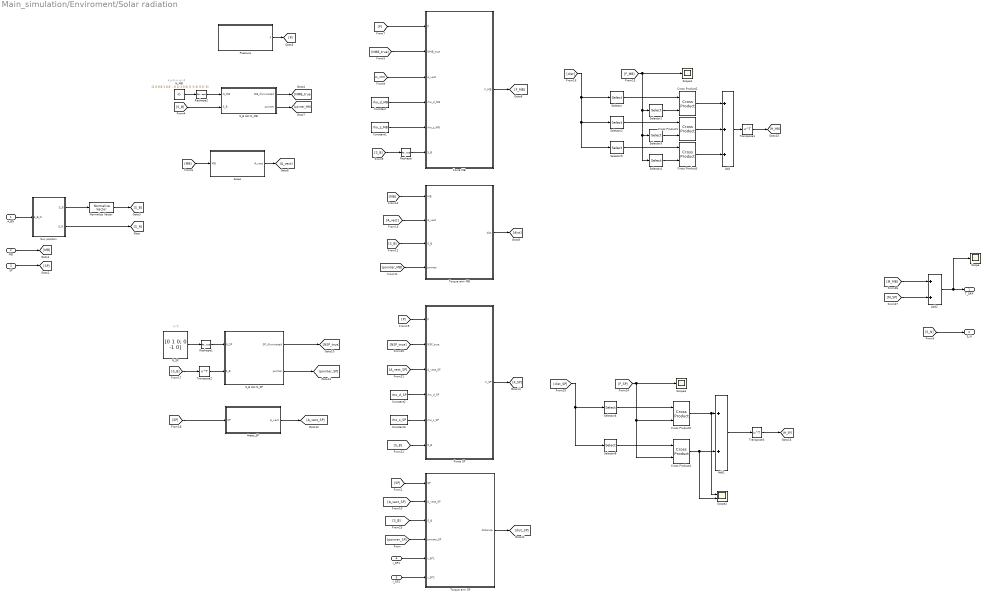
== system Main_simulation/Enviroment/Solar radiation ==
  note: x,y,z,-x,-y,-z
  note: y,-y
  A_BN : Inport
  MB : Inport  Port=2
  SP : Inport  Port=3
  r_SP1 : Inport  Port=4
  r_SP2 : Inport  Port=5
  Add : Sum  Inputs=3
  Add1 : Sum
  Add2 : Sum
  Areas : Subsystem
  Areas_SP : Subsystem
  Constant : Constant  Value=rho_d_MB
  Constant1 : Constant  Value=rho_s_MB
  Constant2 : Constant  Value=rho_d_SP
  Constant3 : Constant  Value=rho_s_SP
  Cross Product{1..5} (5 alike) : matrix_library/Cross Product
      settings: SourceProductBaseCode=SL
  Force MB : Subsystem
  Force SP : Subsystem
  N_MB : Constant  Value=[1 0 0;0 1 0;0 0 1;-1 0 0; 0 -1 0; 0 0 -1]  VectorParams1D=off
  N_SP : Constant  Value=[0 1 0; 0 -1 0]  VectorParams1D=off
  Normalize Vector : vrlib/Utilities/Normalize Vector  maxzero=0
  Pressure : Subsystem
  Reshape : Reshape  OutputDimensionality=Column vector (2-D)
  Reshape1 : Reshape  OutputDimensionality=Customize  OutputDimensions=[2,3]
  Reshape2 : Reshape  OutputDimensionality=Customize  OutputDimensions=[6,3]
  S_B dot N_MB : Subsystem
  S_B dot N_SP : Subsystem
  Scope : Scope
  Scope1 : Scope
  Scope2 : Scope  NumInputPorts=2
  Scope3 : Scope
  Selector : Selector  NumberOfDimensions=2  InputPortWidth=3  IndexOptions=Index vector (dialog),Index vector (dialog)  Indices=1,[1 2 3]  OutputSizes=1,1
  Selector1 : Selector  NumberOfDimensions=2  InputPortWidth=3  IndexOptions=Index vector (dialog),Index vector (dialog)  Indices=1,[1 2 3]  OutputSizes=1,1
  Selector2 : Selector  NumberOfDimensions=2  InputPortWidth=3  IndexOptions=Index vector (dialog),Index vector (dialog)  Indices=2,[1 2 3]  OutputSizes=1,1
  Selector3 : Selector  NumberOfDimensions=2  InputPortWidth=3  IndexOptions=Index vector (dialog),Index vector (dialog)  Indices=2,[1 2 3]  OutputSizes=1,1
  Selector4 : Selector  NumberOfDimensions=2  InputPortWidth=3  IndexOptions=Index vector (dialog),Index vector (dialog)  Indices=3,[1 2 3]  OutputSizes=1,1
  Selector5 : Selector  NumberOfDimensions=2  InputPortWidth=3  IndexOptions=Index vector (dialog),Index vector (dialog)  Indices=3,[1 2 3]  OutputSizes=1,1
  Selector6 : Selector  NumberOfDimensions=2  InputPortWidth=3  IndexOptions=Index vector (dialog),Index vector (dialog)  Indices=1,[1 2 3]  OutputSizes=1,1
  Selector8 : Selector  NumberOfDimensions=2  InputPortWidth=3  IndexOptions=Index vector (dialog),Index vector (dialog)  Indices=2,[1 2 3]  OutputSizes=1,1
  Sun position : Subsystem
  Torque arm MB : Subsystem
  Torque arm SP : Subsystem
  Transpose1 : Math  Operator=transpose  SaturateOnIntegerOverflow=on
  Transpose2 : Math  Operator=transpose  SaturateOnIntegerOverflow=on
  Transpose3 : Math  Operator=transpose  SaturateOnIntegerOverflow=on
  T_SRP : Outport
  S_N : Outport  Port=2
  wires:
  A_BN/1 -> Sun position/1(A_B_N)
  Sun position/1(S_B) -> Normalize Vector/1
  Normalize Vector/1 -> [S_B]
  r_SP1/1 -> Torque arm SP/5(r_SP1)
  r_SP2/1 -> Torque arm SP/6(r_SP2)
  MB/1 -> [MB]
  SP/1 -> [SP]
  Sun position/2(S_N) -> [S_N]
  [S_N] -> S_N/1
  N_MB/1 -> Reshape2/1
  S_B dot N_MB/1(MB_illuminated) -> [NMB_true]
  [NMB_true] -> Force MB/2(NMB_true)
  [S_B] -> S_B dot N_MB/2(S_B)
  [MB] -> Areas/1(MB)
  Pressure/1(P) -> [P]
  Areas/1(A_vect) -> [A_vect]
  [P] -> Force MB/1(P)
  [A_vect] -> Force MB/3(A_vect)
  Constant/1 -> Force MB/4(rho_d_MB)
  Constant1/1 -> Force MB/5(rho_s_MB)
  [S_B] -> Reshape/1
  S_B dot N_MB/2(pointer) -> [pointer_MB]
  [pointer_MB] -> Torque arm MB/4(pointer)
  [S_B] -> Torque arm MB/3(S_B)
  [A_vect] -> Torque arm MB/2(A_vect)
  [MB] -> Torque arm MB/1(MB)
  Reshape/1 -> Force MB/6(S_B)
  Cross Product2/1 -> Add/1
  Selector/1 -> Cross Product2/1
  Selector1/1 -> Cross Product2/2
  Selector3/1 -> Cross Product1/2
  Selector2/1 -> Cross Product1/1
  [dist] -> Selector2/1, Selector5/1, Selector/1
  Cross Product1/1 -> Add/2
  Force MB/1(F_MB) -> [F_MB]
  [F_MB] -> Scope1/1, Selector4/1, Selector3/1, Selector1/1
  Cross Product3/1 -> Add/3
  Selector4/1 -> Cross Product3/2
  Selector5/1 -> Cross Product3/1
  Add/1 -> Transpose1/1
  Torque arm MB/1(dist) -> [dist]
  S_B dot N_SP/2(pointer) -> [pointer_SP]
  Areas_SP/1(A_vect) -> [A_vect_SP]
  [SP] -> Areas_SP/1(SP)
  Transpose2/1 -> S_B dot N_SP/2(S_B)
  [S_B] -> Transpose2/1
  S_B dot N_SP/1(SP_illuminated) -> [NSP_true]
  N_SP/1 -> Reshape1/1
  Reshape1/1 -> S_B dot N_SP/1(N_SP)
  Reshape2/1 -> S_B dot N_MB/1(N_MB)
  [P] -> Force SP/1(P)
  [NSP_true] -> Force SP/2(NSP_true)
  [A_vect_SP] -> Force SP/3(A_vect_SP)
  Constant2/1 -> Force SP/4(rho_d_SP)
  Constant3/1 -> Force SP/5(rho_s_SP)
  [S_B] -> Force SP/6(S_B)
  [pointer_SP] -> Torque arm SP/4(pointer_SP)
  [SP] -> Torque arm SP/1(SP)
  [A_vect_SP] -> Torque arm SP/2(A_vect_SP)
  [S_B] -> Torque arm SP/3(S_B)
  Torque arm SP/1(distance) -> [dist_SP]
  Force SP/1(F_SP) -> [F_SP]
  Transpose3/1 -> [M_SP]
  Add1/1 -> Transpose3/1
  Cross Product4/1 -> Scope2/2, Add1/2
  [dist_SP] -> Selector6/1, Selector8/1
  Selector8/1 -> Cross Product4/1
  [F_SP] -> Cross Product5/2, Cross Product4/2, Scope3/1
  Selector6/1 -> Cross Product5/1
  Cross Product5/1 -> Scope2/1, Add1/1
  Transpose1/1 -> [M_MB]
  [M_MB] -> Add2/1
  Add2/1 -> Scope/1, T_SRP/1
  [M_SP] -> Add2/2

== system Main_simulation/Inertia matrix/r_SP ==
  b_SP : Inport
  a_MB : Inport  Port=2
  Constant : Constant  Value=[1 0 0]
  Gain : Gain  Gain=1/2
  Gain1 : Gain  Gain=1/2
  Gain2 : Gain  Gain=-1
  Product : Product
  Reshape : Reshape  OutputDimensionality=Column vector (2-D)
  Sum : Sum
  r_SP1 : Outport
  r_SP2 : Outport  Port=2
  wires:
  Constant/1 -> Reshape/1
  a_MB/1 -> Gain/1
  b_SP/1 -> Gain1/1
  Gain1/1 -> Sum/1
  Gain/1 -> Sum/2
  Reshape/1 -> Product/1
  Sum/1 -> Product/2
  Gain2/1 -> r_SP2/1
  Product/1 -> r_SP1/1, Gain2/1

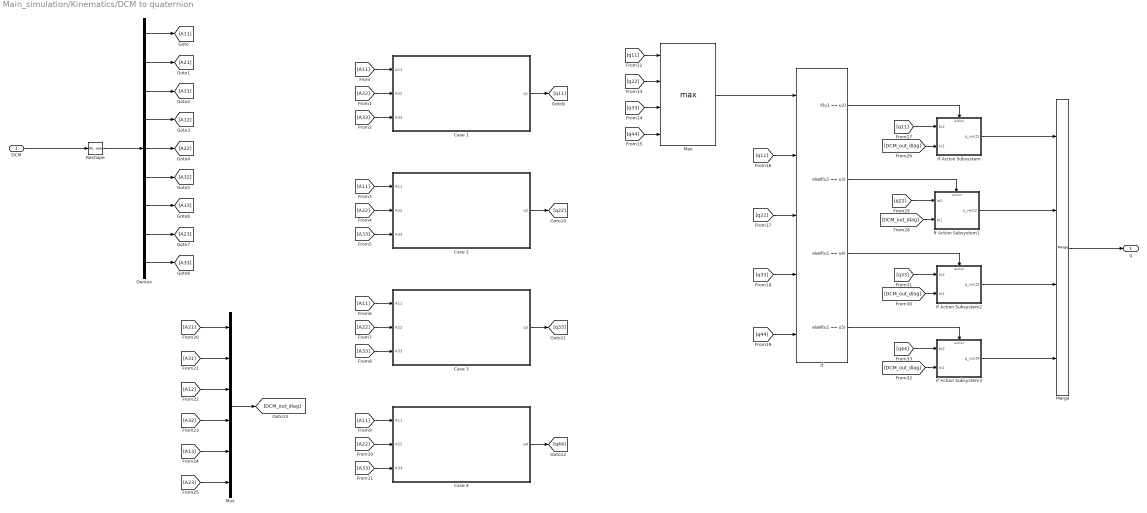
== system Main_simulation/Kinematics/DCM to quaternion ==
  DCM : Inport
  Case 1 : Subsystem
  Case 2 : Subsystem
  Case 3 : Subsystem
  Case 4 : Subsystem
  Demux : Demux  Outputs=9
  If : If  NumInputs=5  IfExpression=u1 == u2  ElseIfExpressions=u1 == u3, u1 == u4, u1 == u5  ShowElse=off
  If Action Subsystem : Subsystem  TreatAsAtomicUnit=on
  If Action Subsystem1 : Subsystem  TreatAsAtomicUnit=on
  If Action Subsystem2 : Subsystem  TreatAsAtomicUnit=on
  If Action Subsystem3 : Subsystem  TreatAsAtomicUnit=on
  Max : MinMax  Function=max  Inputs=4
  Merge : Merge  Inputs=4
  Mux : Mux  Inputs=6
  Reshape : Reshape  OutputDimensionality=Column vector (2-D)
  q : Outport
  wires:
  DCM/1 -> Reshape/1
  Reshape/1 -> Demux/1
  Demux/1 -> [A11]
  Demux/2 -> [A21]
  Demux/3 -> [A31]
  Demux/4 -> [A12]
  Demux/5 -> [A22]
  Demux/6 -> [A32]
  Demux/7 -> [A13]
  Demux/8 -> [A23]
  Demux/9 -> [A33]
  [A22] -> Case 1/2(A22)
  [A33] -> Case 1/3(A33)
  [A11] -> Case 1/1(A11)
  [A11] -> Case 2/1(A11)
  [A33] -> Case 2/3(A33)
  [A22] -> Case 2/2(A22)
  [A22] -> Case 3/2(A22)
  [A33] -> Case 3/3(A33)
  [A11] -> Case 3/1(A11)
  [A11] -> Case 4/1(A11)
  [A33] -> Case 4/3(A33)
  [A22] -> Case 4/2(A22)
  Case 1/1(q1) -> [q11]
  Case 2/1(q2) -> [q22]
  Case 3/1(q3) -> [q33]
  Case 4/1(q4) -> [q44]
  [q11] -> Max/1
  [q33] -> Max/3
  [q22] -> Max/2
  [q44] -> Max/4
  Max/1 -> If/1
  [q11] -> If/2
  [q22] -> If/3
  [q33] -> If/4
  [q44] -> If/5
  If/1 -> If Action Subsystem/Action
  If/2 -> If Action Subsystem1/Action
  If/3 -> If Action Subsystem2/Action
  If/4 -> If Action Subsystem3/Action
  If Action Subsystem3/1(q_vect4) -> Merge/4
  If Action Subsystem2/1(q_vect3) -> Merge/3
  If Action Subsystem1/1(q_vect2) -> Merge/2
  If Action Subsystem/1(q_vect1) -> Merge/1
  Merge/1 -> q/1
  [A23] -> Mux/6
  [A13] -> Mux/5
  [A32] -> Mux/4
  [A12] -> Mux/3
  [A31] -> Mux/2
  [A21] -> Mux/1
  Mux/1 -> [DCM_out_diag]
  [DCM_out_diag] -> If Action Subsystem/2(In1)
  [q11] -> If Action Subsystem/1(In2)
  [q22] -> If Action Subsystem1/1(In2)
  [DCM_out_diag] -> If Action Subsystem1/2(In1)
  [DCM_out_diag] -> If Action Subsystem2/2(In1)
  [q33] -> If Action Subsystem2/1(In2)
  [q44] -> If Action Subsystem3/1(In2)
  [DCM_out_diag] -> If Action Subsystem3/2(In1)

== system Main_simulation/Kinematics/Normalisation ==
  In1 : Inport
  Normalize Vector : vrlib/Utilities/Normalize Vector  maxzero=0
  Reshape : Reshape  OutputDimensionality=Column vector (2-D)
  Out1 : Outport
  wires:
  In1/1 -> Normalize Vector/1
  Normalize Vector/1 -> Reshape/1
  Reshape/1 -> Out1/1

== system Main_simulation/Kinematics/Subsystem ==
  w_B : Inport
  Demux : Demux  Outputs=3
  Gain{1..6} (6 alike) : Gain  Gain=-1
  Ground : Ground
  Reshape : Reshape  OutputDimensionality=Customize  OutputDimensions=[4,4]
  Vector Concatenate : Concatenate  NumInputs=16
  OMEGA : Outport
  wires:
  Ground/1 -> Vector Concatenate/1, Vector Concatenate/6, Vector Concatenate/11, Vector Concatenate/16
  Gain3/1 -> Vector Concatenate/8
  Gain2/1 -> Vector Concatenate/7
  Gain5/1 -> Vector Concatenate/12
  Vector Concatenate/1 -> Reshape/1
  Gain4/1 -> Vector Concatenate/9
  w_B/1 -> Demux/1
  Demux/1 -> [w_Bx]
  Demux/2 -> [w_By]
  Demux/3 -> [w_Bz]
  [w_By] -> Vector Concatenate/3
  Gain6/1 -> Vector Concatenate/4
  Gain1/1 -> Vector Concatenate/2
  [w_Bz] -> Gain1/1
  [w_Bx] -> Gain6/1
  [w_Bz] -> Vector Concatenate/5
  [w_Bx] -> Gain2/1
  [w_By] -> Gain3/1
  [w_By] -> Gain4/1
  [w_Bx] -> Vector Concatenate/10
  [w_Bz] -> Gain5/1
  [w_Bx] -> Vector Concatenate/13
  [w_By] -> Vector Concatenate/14
  [w_Bz] -> Vector Concatenate/15
  Reshape/1 -> [OMEGA]
  [OMEGA] -> OMEGA/1

== system Main_simulation/Kinematics/q to DCM ==
  q_BN : Inport
  Add : Sum  Inputs=+++
  Add1 : Sum  Inputs=+-
  Constant : Constant  Value=[1 0 0; 0 1 0; 0 0 1]
  Demux : Demux
  Gain : Gain  Gain=2
  Matrix Multiply : Product  Multiplication=Matrix(*)
  Matrix Multiply1 : Product  Multiplication=Matrix(*)
  Product : Product
  Product1 : Product
  Reshape : Reshape  OutputDimensionality=Customize  OutputDimensions=[3,3]
  Square : Math  Operator=square  SaturateOnIntegerOverflow=on
  Transpose : Math  Operator=transpose  SaturateOnIntegerOverflow=on
  Transpose1 : Math  Operator=transpose  SaturateOnIntegerOverflow=on
  Vector Concatenate : Concatenate  NumInputs=3
  q cross : Subsystem
  A_BN : Outport
  wires:
  q_BN/1 -> Demux/1
  Demux/1 -> [q1]
  Demux/2 -> [q2]
  Demux/3 -> [q3]
  Demux/4 -> [q4]
  [A_BN1] -> Add/1
  [A_BN2] -> Add/2
  [A_BN3] -> Add/3
  Add/1 -> A_BN/1
  [q1] -> Vector Concatenate/1
  [q2] -> Vector Concatenate/2
  [q3] -> Vector Concatenate/3
  Vector Concatenate/1 -> [q_vec]
  [q4] -> Square/1
  Square/1 -> Add1/1
  [q_vec] -> Transpose/1
  Matrix Multiply/1 -> Add1/2
  Transpose/1 -> Matrix Multiply/1
  [q_vec] -> Matrix Multiply/2
  Product/1 -> [A_BN1]
  Add1/1 -> Product/1
  Constant/1 -> Reshape/1
  Reshape/1 -> Product/2
  [q_vec] -> Transpose1/1
  [q_vec] -> Matrix Multiply1/1
  Transpose1/1 -> Matrix Multiply1/2
  Matrix Multiply1/1 -> Gain/1
  Gain/1 -> [A_BN2]
  [q_vec] -> q cross/1(q_vec)
  [q4] -> Product1/1
  q cross/1(q cross) -> Product1/2
  Product1/1 -> [A_BN3]

== system Main_simulation/Orbit propagation/vector ==
  theta : Inport
  Constant : Constant  Value=i
  Cos : Trigonometry  Operator=cos
  Cos1 : Trigonometry
  Cos2 : Trigonometry  Operator=cos
  Cos3 : Trigonometry
  Cos4 : Trigonometry
  Mux : Mux  Inputs=3
  Product : Product
  Product1 : Product
  Vector : Outport
  wires:
  Mux/1 -> Vector/1
  Cos/1 -> Mux/1
  Cos1/1 -> Product/1
  Cos2/1 -> Product/2
  Product/1 -> Mux/2
  Cos4/1 -> Product1/2
  Product1/1 -> Mux/3
  Cos3/1 -> Product1/1
  theta/1 -> Cos3/1, Cos1/1, Cos/1
  Constant/1 -> Cos4/1, Cos2/1

== system Main_simulation/Relative attitude/A_LN ==
  theta : Inport
  i : Inport  Port=2
  MatrixMultiply : Product  Multiplication=Matrix(*)
  inclination matrix : Subsystem
  true anomaly matrix : Subsystem
  A_L_N : Outport
  wires:
  theta/1 -> true anomaly matrix/1(theta)
  true anomaly matrix/1(M(theta)) -> MatrixMultiply/1
  inclination matrix/1(M(i)) -> MatrixMultiply/2
  MatrixMultiply/1 -> A_L_N/1
  i/1 -> inclination matrix/1(i)

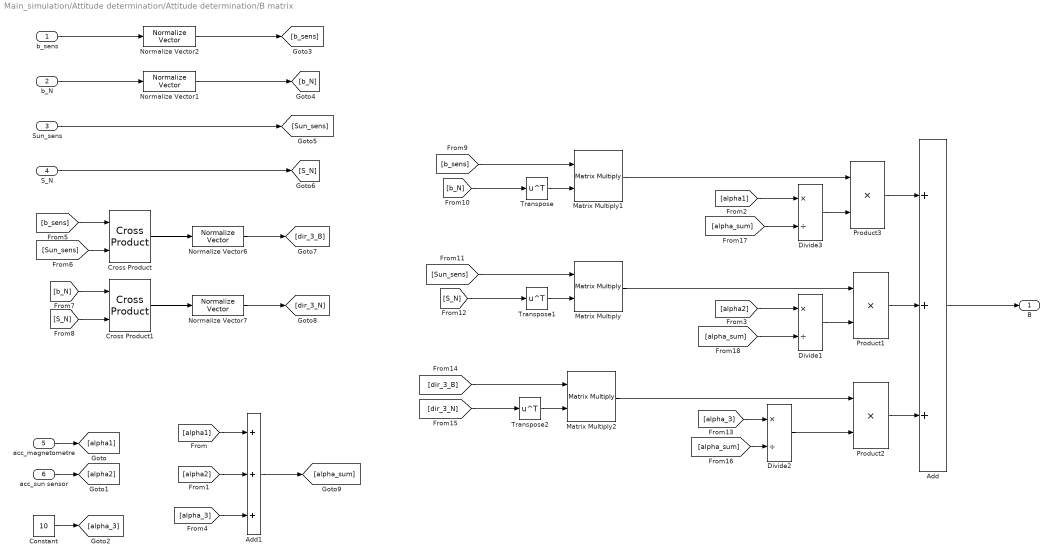
== system Main_simulation/Attitude determination/Attitude determination/B matrix ==
  b_sens : Inport
  b_N : Inport  Port=2
  Sun_sens : Inport  Port=3
  S_N : Inport  Port=4
  acc_magnetometre : Inport  Port=5
  acc_sun sensor : Inport  Port=6
  Add : Sum  Inputs=+++
  Add1 : Sum  Inputs=+++
  Constant : Constant  Value=10
  Cross Product : matrix_library/Cross Product
      settings: SourceProductBaseCode=SL
  Cross Product1 : matrix_library/Cross Product
      settings: SourceProductBaseCode=SL
  Divide1 : Product  Inputs=*/
  Divide2 : Product  Inputs=*/
  Divide3 : Product  Inputs=*/
  Matrix Multiply : Product  Multiplication=Matrix(*)
  Matrix Multiply1 : Product  Multiplication=Matrix(*)
  Matrix Multiply2 : Product  Multiplication=Matrix(*)
  Normalize Vector{1..2,6..7} (4 alike) : vrlib/Utilities/Normalize Vector  maxzero=0
  Product1 : Product
  Product2 : Product
  Product3 : Product
  Transpose : Math  Operator=transpose  SaturateOnIntegerOverflow=on
  Transpose1 : Math  Operator=transpose  SaturateOnIntegerOverflow=on
  Transpose2 : Math  Operator=transpose  SaturateOnIntegerOverflow=on
  B : Outport
  wires:
  Transpose/1 -> Matrix Multiply1/2
  [b_sens] -> Matrix Multiply1/1
  Add/1 -> B/1
  [alpha1] -> Add1/1
  Transpose1/1 -> Matrix Multiply/2
  acc_sun sensor/1 -> [alpha2]
  [alpha2] -> Add1/2
  acc_magnetometre/1 -> [alpha1]
  [b_N] -> Transpose/1
  Constant/1 -> [alpha_3]
  [alpha_3] -> Add1/3
  b_sens/1 -> Normalize Vector2/1
  [b_sens] -> Cross Product/1
  [Sun_sens] -> Cross Product/2
  [S_N] -> Cross Product1/2
  [b_N] -> Cross Product1/1
  Cross Product/1 -> Normalize Vector6/1
  Cross Product1/1 -> Normalize Vector7/1
  Normalize Vector2/1 -> [b_sens]
  b_N/1 -> Normalize Vector1/1
  Sun_sens/1 -> [Sun_sens]
  S_N/1 -> [S_N]
  Normalize Vector6/1 -> [dir_3_B]
  Normalize Vector7/1 -> [dir_3_N]
  [Sun_sens] -> Matrix Multiply/1
  [S_N] -> Transpose1/1
  Product2/1 -> Add/3
  Divide2/1 -> Product2/2
  [alpha_3] -> Divide2/1
  [dir_3_N] -> Transpose2/1
  [dir_3_B] -> Matrix Multiply2/1
  Matrix Multiply2/1 -> Product2/1
  Transpose2/1 -> Matrix Multiply2/2
  Add1/1 -> [alpha_sum]
  [alpha_sum] -> Divide2/2
  [alpha1] -> Divide3/1
  [alpha_sum] -> Divide3/2
  [alpha2] -> Divide1/1
  [alpha_sum] -> Divide1/2
  Divide3/1 -> Product3/2
  Matrix Multiply1/1 -> Product3/1
  Product3/1 -> Add/1
  Product1/1 -> Add/2
  Matrix Multiply/1 -> Product1/1
  Divide1/1 -> Product1/2
  Normalize Vector1/1 -> [b_N]

== system Main_simulation/Attitude determination/Attitude determination/If Action Subsystem ==
  In1 : Inport
  Action Port : ActionPort  ActionPortLabel=if(u1 == u5)
  Out1 : Outport
  wires:
  In1/1 -> Out1/1

== system Main_simulation/Attitude determination/Attitude determination/If Action Subsystem1 ==
  In1 : Inport
  Action Port : ActionPort  ActionPortLabel=elseif(u2 == u5)
  Out1 : Outport
  wires:
  In1/1 -> Out1/1

== system Main_simulation/Attitude determination/Attitude determination/If Action Subsystem2 ==
  In1 : Inport
  Action Port : ActionPort  ActionPortLabel=elseif( u3 ==u5)
  Out1 : Outport
  wires:
  In1/1 -> Out1/1

== system Main_simulation/Attitude determination/Attitude determination/If Action Subsystem3 ==
  In1 : Inport
  Action Port : ActionPort  ActionPortLabel=elseif( u4 == u5)
  Out1 : Outport
  wires:
  In1/1 -> Out1/1
